simulink model "YAW_accn"  (R2015a)
settings: Solver=ode45  StartTime=0.0  StopTime=10.0  RelTol=1e-3
undefined symbols (not defined in the file): I_z, l_f, l_r, l_w
settings Model: Creator=BML  LastModifiedBy=BML

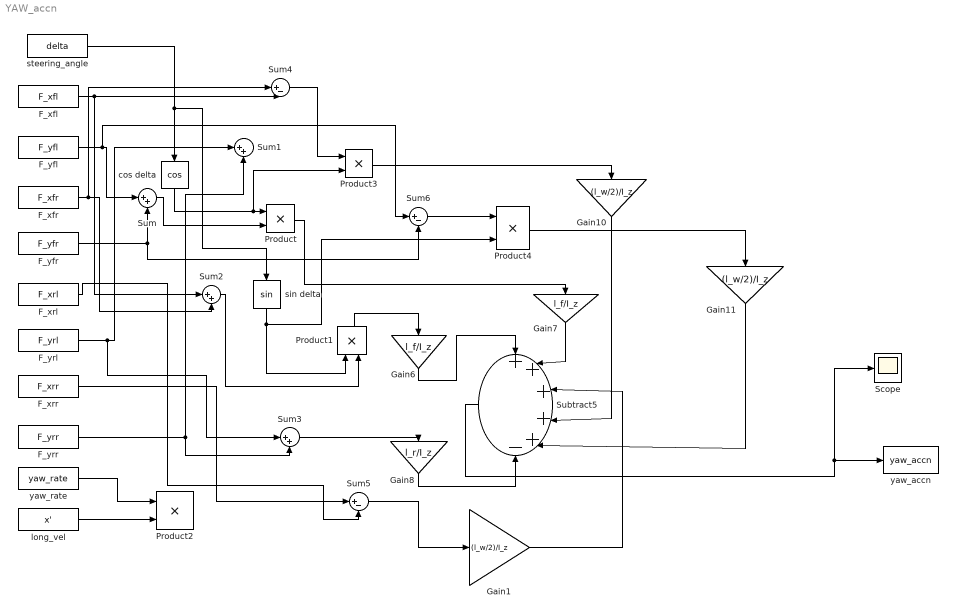
== system YAW_accn ==
  F_xfl : FromWorkspace  VariableName=F_xfl  SampleTime=0
  F_xfr : FromWorkspace  VariableName=F_xfr  SampleTime=0
  F_xrl : FromWorkspace  VariableName=F_xrl  SampleTime=0
  F_xrr : FromWorkspace  VariableName=F_xrr  SampleTime=0
  F_yfl : FromWorkspace  VariableName=F_yfl  SampleTime=0
  F_yfr : FromWorkspace  VariableName=F_yfr  SampleTime=0
  F_yrl : FromWorkspace  VariableName=F_yrl  SampleTime=0
  F_yrr : FromWorkspace  VariableName=F_yrr  SampleTime=0
  Gain1 : Gain  Gain=(l_w/2)/I_z
  Gain10 : Gain  Gain=(l_w/2)/I_z
  Gain11 : Gain  Gain=(l_w/2)/I_z
  Gain6 : Gain  Gain=l_f/I_z
  Gain7 : Gain  Gain=l_f/I_z
  Gain8 : Gain  Gain=l_r/I_z
  Product{,1..4} (5 alike) : Product
  Scope : Scope
  Subtract5 : Sum  Inputs=+++++-
  Sum{,1..3} (4 alike) : Sum  Inputs=|++
  Sum4 : Sum  Inputs=|+-
  Sum5 : Sum  Inputs=|+-
  Sum6 : Sum  Inputs=|+-
  cos delta : Trigonometry  Operator=cos
  long_vel : FromWorkspace  VariableName=x'  SampleTime=0
  "sin delta " : Trigonometry
  steering_angle : FromWorkspace  VariableName=delta  SampleTime=0
  yaw_accn : ToWorkspace  VariableName=yaw_accn  SaveFormat=Timeseries  SampleTime=-1
  yaw_rate : FromWorkspace  VariableName=yaw_rate  SampleTime=0
  wires:
  cos delta/1 -> Product3/2, Product/1
  Sum/1 -> Product/2
  long_vel/1 -> Product2/2
  steering_angle/1 -> "sin delta "/1, cos delta/1
  "sin delta "/1 -> Product4/2, Product1/1
  Sum2/1 -> Product1/2
  yaw_rate/1 -> Product2/1
  F_xfl/1 -> Sum2/1, Sum4/2
  F_xfr/1 -> Sum4/1, Sum2/2
  F_yrl/1 -> Sum3/1, Sum1/1
  F_yfl/1 -> Sum6/1, Sum/1
  F_yfr/1 -> Sum/2, Sum6/2
  Gain10/1 -> Subtract5/4
  Gain11/1 -> Subtract5/5
  Gain6/1 -> Subtract5/1
  Gain8/1 -> Subtract5/6
  Gain7/1 -> Subtract5/2
  Product1/1 -> Gain6/1
  Product/1 -> Gain7/1
  F_yrr/1 -> Sum1/2, Sum3/2
  Sum3/1 -> Gain8/1
  Sum4/1 -> Product3/1
  Product3/1 -> Gain10/1
  F_xrr/1 -> Sum5/1
  F_xrl/1 -> Sum5/2
  Sum5/1 -> Gain1/1
  Gain1/1 -> Subtract5/3
  Sum6/1 -> Product4/1
  Product4/1 -> Gain11/1
  Subtract5/1 -> Scope/1, yaw_accn/1
